simulink model "Third_Impact_final2"  (R2025a)
settings: Solver=ode23tb  StartTime=0  StopTime=1000  FixedStep=Ts  RelTol=1e-3
PostLoadFcn:
  | helperSLHighwayLaneFollowingWithRRSetup()
values from neighbouring files (symbols this model uses):
  numTargetActors = numActors - 1    [helperSLHighwayLaneFollowingWithRRSetup.m]
  vehSim3D = repmat(     struct(     'Length', 0,     'RearOverhang', 0,     'InitialPos',[0 0 0],     'InitialRot',[0 0 0]),     numVehicles,1)    [helperSLHighwayLaneFollowingWithRRSetup.m]
undefined symbols (not defined in the file or in its folder): Defined, des_vel, Ego, genDelta, genTarget, Lane, laneChange, m, n, Ts, User
libraries: sim3dautolib x5, roadrunnerscenario x4, simulink x4, sim3dlib x1
CloseFcn:
  | helperSLHighwayLaneFollowingWithRRCleanUp()
settings Model: SILPILModeSetting=veronly  SILPILSystemUnderTest=refmodels  Creator=The MathWorks, Inc.  LastModifiedBy=leskb
settings SolverCC: AlgebraicLoopSolver=TrustRegion  MaxZcPerStep=1.0
settings DataIOCC: SaveOutput=off  DSMLogging=off  SaveTime=off  ReturnWorkspaceOutputs=off
settings OptimizationCC: ReuseModelBlockBuffer=off
settings DebuggingCC: ParameterPrecisionLossMsg=none  UnconnectedInputMsg=warning  UnconnectedOutputMsg=warning  UnconnectedLineMsg=warning  PregeneratedLibrarySubsystemCodeDiagnostic=none  SubsystemReferenceDiagnosticForUnitTest=warning  ArithmeticOperatorsInVariantConditions=warning
settings HardwareCC: ProdLongLongMode=on
settings ModelReferenceCC: EnableRefExpFcnMdlSchedulingChecks=on
settings SFSimCC: SimUseLocalCustomCode=off
settings RTWCC: RTWUseLocalCustomCode=off  GPUComputeCapability=3.5  DLArmComputeVersion=19.05
settings GRTTargetCC: RTWCAPISignals=on
settings ConfigComp: CovScope=ReferencedModels  CovIncludeTopModel=off

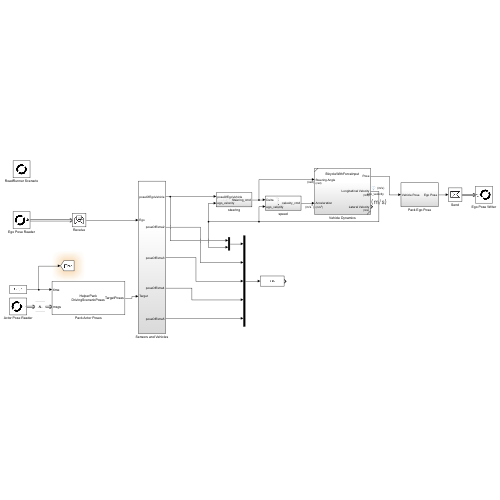
[thumbnail: Simulink's stored preview of the top-level diagram]
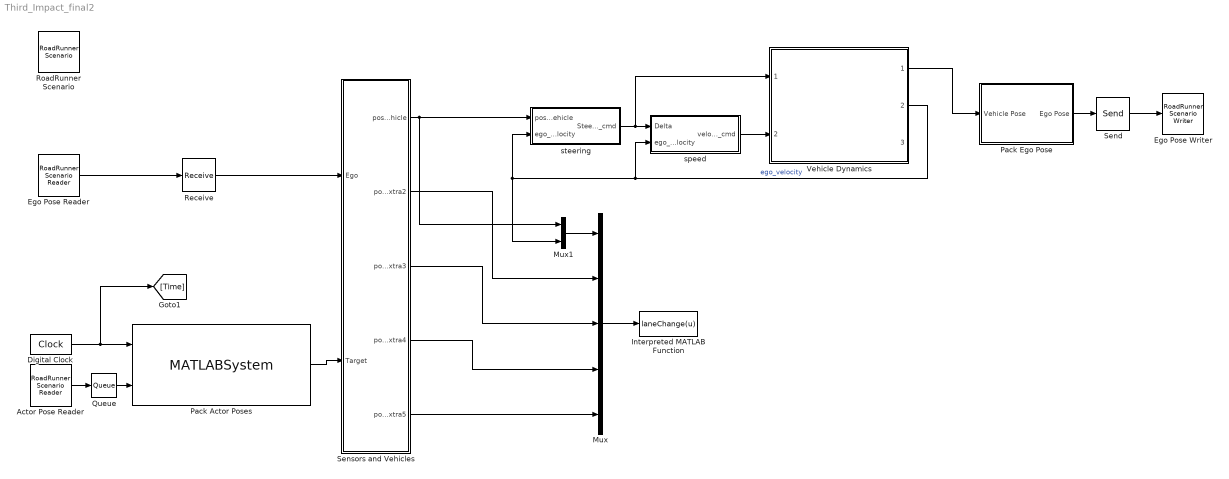
== system Third_Impact_final2 ==
  Actor Pose Reader : roadrunnerscenario/RoadRunner Scenario Reader  TopicCategory=Actor  ActorCategory=All Types  ActionType=Path Following  EventType=User-Defined  TopicType=Actor Pose (Driving Scenario compatible)  VehicleType=Vehicle Specifications  TrafficSignalType=Traffic Signal Specifications  TrafficSignalControllerType=Traffic Signal Controller Specifications  UserDefinedAction=Action1  UserDefinedEvent=Event1  Filter=None  AdditionalRelationship=None  SensorTopic=Target Poses  LaneBoundaryOutputTopic=Ego-Lane  SensorID=1  SampleTime=Ts
  Digital Clock : DigitalClock  SampleTime=Ts
  Ego Pose Reader : roadrunnerscenario/RoadRunner Scenario Reader  TopicCategory=Actor  ActorCategory=All Types  ActionType=Path Following  EventType=User-Defined  TopicType=Actor Pose (Driving Scenario compatible)  VehicleType=Vehicle Specifications  TrafficSignalType=Traffic Signal Specifications  TrafficSignalControllerType=Traffic Signal Controller Specifications  UserDefinedAction=Action1  UserDefinedEvent=Event1  Filter=Self  AdditionalRelationship=None  SensorTopic=Target Poses  LaneBoundaryOutputTopic=Ego-Lane  SensorID=1  SampleTime=Ts
  Ego Pose Writer : roadrunnerscenario/RoadRunner Scenario Writer  TopicCategory=Actor  ActorCategory=All Types  EventType=Action Complete  UserDefinedEvent=Event1  VehicleType=Vehicle Pose  TopicType=Actor Pose (Driving Scenario compatible)
  Interpreted MATLAB Function : MATLABFcn  MATLABFcn=laneChange(u)
  Mux : Mux  Inputs=[4 4 4 4 4]
  Mux1 : Mux  Inputs=2
  Pack Actor Poses : MATLABSystem  InputPortMessageModes=n,m  System=HelperPackDrivingScenarioPoses  EgoActorID=1  ActorProfiles=actorProfiles  DefaultActorPoses="Simulink.Bus.createMATLABStruct( \"BusActors\" )"
      mask Type: HelperPackDrivingScenarioPoses
  Pack Ego Pose : Subsystem
  Queue : Queue  InputPortMessageModes=m  OutputPortMessageModes=m  OverwriteOldest=on  Capacity=numTargetActors+2  QueueType=LIFO
  Receive : Receive  InputPortMessageModes=m  UseInternalQueue=off  QueueOverwriting=on  QueueLength=1  QueueType=LIFO  SampleTime=Ts
  RoadRunner Scenario : roadrunnerscenario/RoadRunner Scenario  UserDefinedActions={}  UserDefinedEvents={}  PathPoints=500
  Send : Send  OutputPortMessageModes=m
  Sensors and Vehicles : Subsystem  VariantControl=1
  Vehicle Dynamics : Subsystem  VariantControl=Variant2  ReferencedSubsystem=BicycleWithForceInput
  speed : Subsystem
  steering : Subsystem
  wires:
  Ego Pose Reader/1 -> Receive/1
  Digital Clock/1 -> Pack Actor Poses/1, [Time]
  Send/1 -> Ego Pose Writer/1
  Vehicle Dynamics/1 -> Pack Ego Pose/1(Vehicle Pose)
  Receive/1 -> Sensors and Vehicles/1(Ego)
  Actor Pose Reader/1 -> Queue/1
  Pack Ego Pose/1(Ego Pose) -> Send/1
  Queue/1 -> Pack Actor Poses/2
  Pack Actor Poses/1 -> Sensors and Vehicles/2(Target)
  Vehicle Dynamics/2 -> speed/2(ego_velocity), steering/2(ego_velocity), Mux1/2  "ego_velocity"
  speed/1(velocity_cmd) -> Vehicle Dynamics/2
  steering/1(Steering_cmd) -> speed/1(Delta), Vehicle Dynamics/1
  Sensors and Vehicles/1(poseOfEgoVehicle) -> Mux1/1, steering/1(poseOfEgoVehicle)
  Sensors and Vehicles/2(poseOfExtra2) -> Mux/2
  Sensors and Vehicles/3(poseOfExtra3) -> Mux/3
  Sensors and Vehicles/4(poseOfExtra4) -> Mux/4
  Sensors and Vehicles/5(poseOfExtra5) -> Mux/5
  Mux/1 -> Interpreted MATLAB Function/1
  Mux1/1 -> Mux/1

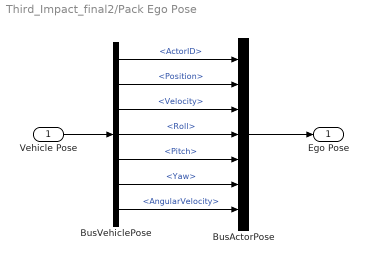
== system Third_Impact_final2/Pack Ego Pose ==
  Vehicle Pose : Inport
  BusActorPose : BusCreator  Inputs=7  OutDataTypeStr=Bus: BusActorPose  NonVirtualBus=on
      settings: InheritFromInputs=off
  BusVehiclePose : BusSelector  OutputSignals=ActorID,Position,Velocity,Roll,Pitch,Yaw,AngularVelocity
  Ego Pose : Outport
  wires:
  BusVehiclePose/4 -> BusActorPose/4  "<Roll>"
  BusVehiclePose/3 -> BusActorPose/3  "<Velocity>"
  BusVehiclePose/1 -> BusActorPose/1  "<ActorID>"
  BusVehiclePose/2 -> BusActorPose/2  "<Position>"
  BusVehiclePose/7 -> BusActorPose/7  "<AngularVelocity>"
  BusVehiclePose/6 -> BusActorPose/6  "<Yaw>"
  BusVehiclePose/5 -> BusActorPose/5  "<Pitch>"
  Vehicle Pose/1 -> BusVehiclePose/1
  BusActorPose/1 -> Ego Pose/1

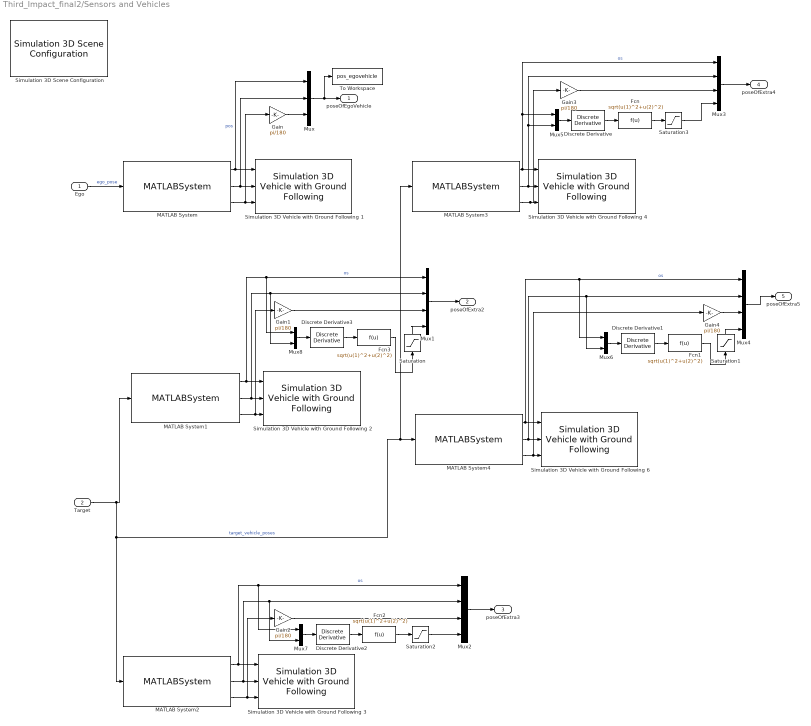
== system Third_Impact_final2/Sensors and Vehicles ==
  Ego : Inport
  Target : Inport  Port=2
  Discrete Derivative{,1..3} (4 alike) : simulink/Discrete/Discrete Derivative  gainval=1.0  ICPrevScaledInput=0.0  OutMin=[]  OutMax=[]  OutDataType=fixdt(1, 16)  OutScaling=2^-10  DoSatur=off
  Fcn{,1..3} (4 alike) : Fcn  Expr=sqrt(u(1)^2+u(2)^2)
  Gain{,1..4} (5 alike) : Gain  Gain=pi/180
  MATLAB System : MATLABSystem  System=HelperConvertDSPoseToSim3D  ActorProfiles=actorProfiles  ActorIDToConvert=1  SimulateUsing=Interpreted execution
      mask Type: HelperConvertDSPoseToSim3D
  MATLAB System1 : MATLABSystem  System=HelperConvertDSPoseToSim3D  ActorProfiles=actorProfiles  ActorIDToConvert=2  SimulateUsing=Interpreted execution
      mask Type: HelperConvertDSPoseToSim3D
  MATLAB System2 : MATLABSystem  System=HelperConvertDSPoseToSim3D  ActorProfiles=actorProfiles  ActorIDToConvert=3  SimulateUsing=Interpreted execution
      mask Type: HelperConvertDSPoseToSim3D
  MATLAB System3 : MATLABSystem  System=HelperConvertDSPoseToSim3D  ActorProfiles=actorProfiles  ActorIDToConvert=4  SimulateUsing=Interpreted execution
      mask Type: HelperConvertDSPoseToSim3D
  MATLAB System4 : MATLABSystem  System=HelperConvertDSPoseToSim3D  ActorProfiles=actorProfiles  ActorIDToConvert=5  SimulateUsing=Interpreted execution
      mask Type: HelperConvertDSPoseToSim3D
  Mux : Mux  Inputs=3
  Mux{1..4} (4 alike) : Mux
  Mux{5..8} (4 alike) : Mux  Inputs=2
  Saturation{,1..3} (4 alike) : Saturate  UpperLimit=100  LowerLimit=-100
  Simulation 3D Scene Configuration : sim3dlib/Simulation 3D Scene Configuration  Priority=0  ProjectFormat=Default Scenes  SceneDesc=Straight road  ProjectName=C:\Program Files\MATLAB\R2025a\toolbox\shared\sim3d_projects\automotive_project_windows\UE\WindowsNoEditor\VehicleSimulation.exe  ScenePath=/Game/Maps/HwStrght  EnableOpenDRIVE=off  vehTagList={'Custom';'Scene Origin';'SimulinkVehicle1';'SimulinkVehicle2';'SimulinkVehicle4';'SimulinkVehicle5';'SimulinkVehicle6'}  vehTag=SimulinkVehicle1  AttachedCameraRelativeTranslation=[0 0 0]  FreeCameraDefaultInitialTranslation=[-6, 0, 2]  AttachedCameraRelativeRotation=[0 0 0]  FreeCameraDefaultInitialRotation=[0, -15, 0]  ViewpointName=Custom  FreeCameraInitialTranslation=[0, 0, 0]  ViewpointTranslation=[0 0 0]  FreeCameraInitialRotation=[0, 0, 0]  ViewpointRotation=[0 0 0]  OpVisEn=off  Ts=Ts  EnableWindow=off  EnableRemoteAccess=off  EnableWeather=off  SunAzimuth=90  SunAltitude=40.0  EnableGeospatialSun=off  Latitude=0  Longitude=0  Date=2023-01-01  Time=10:30:00  GeoTimeZone=-5.0  SunDaylightSaving=off  wind=1  clouds=10  EnableVolumetricClouds=off  CloudCoverage=0  CloudAltitude=6  fog=0  rain=0  RaindropsEffect=off  SnowDensity=0  EnableGeospatial=off  TilesetSource=Earth terrain  UseTrueOrigin=off  OriginHeight=200  OriginLatitude=40.744652  OriginLongitude=-73.988864  MapStyle=Aerial  AdditionalAssetIDs=[]  UseAdvancedSunSky=off  SolarTime=11  TimeZone=-5  Day=21  Month=9  Year=2022  UseDaylightSavingTime=on  DSTStartDay=10  DSTStartMonth=3  DSTEndDay=3  DSTEndMonth=11  DSTSwitchHour=2  sensorTag=MainCamera3  sensorId=3  sensorName=MainCamera3  mountLoc=Origin  offsetFlag=off  tmountOffset=[0, 0, 0]  rmountOffset=[0, 0, 0]  HorizontalResolution=1280  VerticalResolution=720  HorizontalFOV=60  mountPoint=[0 0 0]  mountOrientation=[0 0 0]  aMode=3  ID=3  GeoTrigger=Inactive  ViewNameList={'Custom'}  ViewTranslationList={'[0 0 0]'}  ViewRotationList={'[0 0 0]'}
      settings: LibrarySourceBlock=drivingsim3d/Simulation 3D Scene Configuration
  Simulation 3D Vehicle with Ground Following 1 : sim3dautolib/Simulation 3D Vehicle with Ground Following  Priority=-1  PassVehMesh=Sedan  MeshPath=/MathWorksSimulation/Vehicles/Muscle/Meshes/SK_MuscleCar.SK_MuscleCar  TrackWidth=1.9  WheelBase=3  WheelRadius=0.35  VehColor=Blue  CoordinateSystem=ISO8855  InitialPos=vehSim3D(1).InitialPos  InitialRot=vehSim3D(1).InitialRot  ActorName=SimulinkVehicle1  SampleTime=-1  ActorType=SimulinkVehicle  ID=1  aMode=3  ActorTag=SimulinkVehicle1  CoordinateScheme=ISO  VehLightsControl=off  HeadlightColor=[ 1, 1, 1 ]  HighBeamIntensity=100000  LowBeamIntensity=60000  HighBeamConeAngle=70  LowBeamConeAngle=70  LeftHeadlightOrientation=[ 0, 0 ]  RightHeadlightOrientation=[ 0, 0 ]  BrakelightIntensity=500  ReverselightIntensity=500  SignallightIntensity=500  SignallightPeriod=1  SignalPulseWidth=50  TransformOutportEnabled=off
      settings: LibrarySourceBlock=drivingsim3d/Simulation 3D Vehicle with Ground Following
      settings: AttributesFormatString=|
      | --------------------------------------
      | ActorName = %<ActorName>
      | PassVehMesh = %<PassVehMesh>
      | VehColor = %<VehColor>
      | InitialPos = %<InitialPos>
      | InitialRot = %<InitialRot>
      | Priority = %<Priority>
  Simulation 3D Vehicle with Ground Following 2 : sim3dautolib/Simulation 3D Vehicle with Ground Following  Priority=-1  PassVehMesh=Sedan  MeshPath=/MathWorksSimulation/Vehicles/Muscle/Meshes/SK_MuscleCar.SK_MuscleCar  TrackWidth=1.9  WheelBase=3  WheelRadius=0.35  VehColor=Red  CoordinateSystem=ISO8855  InitialPos=vehSim3D(2).InitialPos  InitialRot=vehSim3D(2).InitialRot  ActorName=SimulinkVehicle2  SampleTime=-1  ActorType=SimulinkVehicle  ID=2  aMode=3  ActorTag=SimulinkVehicle2  CoordinateScheme=ISO  VehLightsControl=off  HeadlightColor=[ 1, 1, 1 ]  HighBeamIntensity=100000  LowBeamIntensity=60000  HighBeamConeAngle=70  LowBeamConeAngle=70  LeftHeadlightOrientation=[ 0, 0 ]  RightHeadlightOrientation=[ 0, 0 ]  BrakelightIntensity=500  ReverselightIntensity=500  SignallightIntensity=500  SignallightPeriod=1  SignalPulseWidth=50  TransformOutportEnabled=off
      settings: LibrarySourceBlock=drivingsim3d/Simulation 3D Vehicle with Ground Following
      settings: AttributesFormatString=|
      | --------------------------------------
      | ActorName = %<ActorName>
      | PassVehMesh = %<PassVehMesh>
      | VehColor = %<VehColor>
      | InitialPos = %<InitialPos>
      | InitialRot = %<InitialRot>
      | Priority = %<Priority>
  Simulation 3D Vehicle with Ground Following 3 : sim3dautolib/Simulation 3D Vehicle with Ground Following  Priority=-1  PassVehMesh=Sedan  MeshPath=/MathWorksSimulation/Vehicles/Muscle/Meshes/SK_MuscleCar.SK_MuscleCar  TrackWidth=1.9  WheelBase=3  WheelRadius=0.35  VehColor=Black  CoordinateSystem=ISO8855  InitialPos=vehSim3D(3).InitialPos  InitialRot=vehSim3D(3).InitialRot  ActorName=SimulinkVehicle4  SampleTime=-1  ActorType=SimulinkVehicle  ID=4  aMode=3  ActorTag=SimulinkVehicle4  CoordinateScheme=ISO  VehLightsControl=off  HeadlightColor=[ 1, 1, 1 ]  HighBeamIntensity=100000  LowBeamIntensity=60000  HighBeamConeAngle=70  LowBeamConeAngle=70  LeftHeadlightOrientation=[ 0, 0 ]  RightHeadlightOrientation=[ 0, 0 ]  BrakelightIntensity=500  ReverselightIntensity=500  SignallightIntensity=500  SignallightPeriod=1  SignalPulseWidth=50  TransformOutportEnabled=off
      settings: LibrarySourceBlock=drivingsim3d/Simulation 3D Vehicle with Ground Following
      settings: AttributesFormatString=|
      | --------------------------------------
      | ActorName = %<ActorName>
      | PassVehMesh = %<PassVehMesh>
      | VehColor = %<VehColor>
      | InitialPos = %<InitialPos>
      | InitialRot = %<InitialRot>
      | Priority = %<Priority>
  Simulation 3D Vehicle with Ground Following 4 : sim3dautolib/Simulation 3D Vehicle with Ground Following  Priority=-1  PassVehMesh=Sedan  MeshPath=/MathWorksSimulation/Vehicles/Muscle/Meshes/SK_MuscleCar.SK_MuscleCar  TrackWidth=1.9  WheelBase=3  WheelRadius=0.35  VehColor=Orange  CoordinateSystem=ISO8855  InitialPos=vehSim3D(4).InitialPos  InitialRot=vehSim3D(4).InitialRot  ActorName=SimulinkVehicle5  SampleTime=-1  ActorType=SimulinkVehicle  ID=5  aMode=3  ActorTag=SimulinkVehicle5  CoordinateScheme=ISO  VehLightsControl=off  HeadlightColor=[ 1, 1, 1 ]  HighBeamIntensity=100000  LowBeamIntensity=60000  HighBeamConeAngle=70  LowBeamConeAngle=70  LeftHeadlightOrientation=[ 0, 0 ]  RightHeadlightOrientation=[ 0, 0 ]  BrakelightIntensity=500  ReverselightIntensity=500  SignallightIntensity=500  SignallightPeriod=1  SignalPulseWidth=50  TransformOutportEnabled=off
      settings: LibrarySourceBlock=drivingsim3d/Simulation 3D Vehicle with Ground Following
      settings: AttributesFormatString=|
      | --------------------------------------
      | ActorName = %<ActorName>
      | PassVehMesh = %<PassVehMesh>
      | VehColor = %<VehColor>
      | InitialPos = %<InitialPos>
      | InitialRot = %<InitialRot>
      | Priority = %<Priority>
  Simulation 3D Vehicle with Ground Following 6 : sim3dautolib/Simulation 3D Vehicle with Ground Following  Priority=-1  PassVehMesh=Sedan  MeshPath=/MathWorksSimulation/Vehicles/Muscle/Meshes/SK_MuscleCar.SK_MuscleCar  TrackWidth=1.9  WheelBase=3  WheelRadius=0.35  VehColor=Green  CoordinateSystem=ISO8855  InitialPos=vehSim3D(5).InitialPos  InitialRot=vehSim3D(5).InitialRot  ActorName=SimulinkVehicle6  SampleTime=-1  ActorType=SimulinkVehicle  ID=6  aMode=3  ActorTag=SimulinkVehicle6  CoordinateScheme=ISO  VehLightsControl=off  HeadlightColor=[ 1, 1, 1 ]  HighBeamIntensity=100000  LowBeamIntensity=60000  HighBeamConeAngle=70  LowBeamConeAngle=70  LeftHeadlightOrientation=[ 0, 0 ]  RightHeadlightOrientation=[ 0, 0 ]  BrakelightIntensity=500  ReverselightIntensity=500  SignallightIntensity=500  SignallightPeriod=1  SignalPulseWidth=50  TransformOutportEnabled=off
      settings: LibrarySourceBlock=drivingsim3d/Simulation 3D Vehicle with Ground Following
      settings: AttributesFormatString=|
      | --------------------------------------
      | ActorName = %<ActorName>
      | PassVehMesh = %<PassVehMesh>
      | VehColor = %<VehColor>
      | InitialPos = %<InitialPos>
      | InitialRot = %<InitialRot>
      | Priority = %<Priority>
  To Workspace : ToWorkspace  VariableName=pos_egovehicle  SaveFormat=Timeseries  SampleTime=-1
  poseOfEgoVehicle : Outport
  poseOfExtra2 : Outport  Port=2
  poseOfExtra3 : Outport  Port=3
  poseOfExtra4 : Outport  Port=4
  poseOfExtra5 : Outport  Port=5
  wires:
  MATLAB System/2 -> Mux/2, Simulation 3D Vehicle with Ground Following 1/2
  MATLAB System/1 -> Mux/1, Simulation 3D Vehicle with Ground Following 1/1  "pos"
  MATLAB System/3 -> Gain/1, Simulation 3D Vehicle with Ground Following 1/3
  Ego/1 -> MATLAB System/1  "ego_pose"
  Target/1 -> MATLAB System2/1, MATLAB System4/1, MATLAB System3/1, MATLAB System1/1  "target_vehicle_poses"
  Mux/1 -> To Workspace/1, poseOfEgoVehicle/1
  Gain/1 -> Mux/3
  Gain1/1 -> Mux1/3
  Mux1/1 -> poseOfExtra2/1
  MATLAB System1/3 -> Gain1/1, Simulation 3D Vehicle with Ground Following 2/3
  MATLAB System2/3 -> Gain2/1, Simulation 3D Vehicle with Ground Following 3/3
  Gain2/1 -> Mux2/3
  Mux2/1 -> poseOfExtra3/1
  MATLAB System3/3 -> Gain3/1, Simulation 3D Vehicle with Ground Following 4/3
  MATLAB System3/1 -> Mux5/1, Mux3/1, Simulation 3D Vehicle with Ground Following 4/1  "os"
  Mux3/1 -> poseOfExtra4/1
  Gain3/1 -> Mux3/3
  MATLAB System3/2 -> Mux5/2, Mux3/2, Simulation 3D Vehicle with Ground Following 4/2
  Gain4/1 -> Mux4/3
  Mux4/1 -> poseOfExtra5/1
  MATLAB System4/3 -> Gain4/1, Simulation 3D Vehicle with Ground Following 6/3
  MATLAB System4/2 -> Mux4/2, Mux6/2, Simulation 3D Vehicle with Ground Following 6/2
  Mux5/1 -> Discrete Derivative/1
  Discrete Derivative/1 -> Fcn/1
  Fcn/1 -> Saturation3/1
  Mux6/1 -> Discrete Derivative1/1
  Discrete Derivative1/1 -> Fcn1/1
  MATLAB System4/1 -> Mux4/1, Mux6/1, Simulation 3D Vehicle with Ground Following 6/1  "os"
  Fcn1/1 -> Saturation1/1
  MATLAB System2/2 -> Mux7/2, Mux2/2, Simulation 3D Vehicle with Ground Following 3/2
  Mux7/1 -> Discrete Derivative2/1
  Discrete Derivative2/1 -> Fcn2/1
  MATLAB System2/1 -> Mux7/1, Mux2/1, Simulation 3D Vehicle with Ground Following 3/1  "os"
  Fcn2/1 -> Saturation2/1
  MATLAB System1/2 -> Mux1/2, Mux8/2, Simulation 3D Vehicle with Ground Following 2/2
  Mux8/1 -> Discrete Derivative3/1
  Discrete Derivative3/1 -> Fcn3/1
  MATLAB System1/1 -> Mux8/1, Mux1/1, Simulation 3D Vehicle with Ground Following 2/1  "os"
  Fcn3/1 -> Saturation/1
  Saturation/1 -> Mux1/4
  Saturation1/1 -> Mux4/4
  Saturation2/1 -> Mux2/4
  Saturation3/1 -> Mux3/4

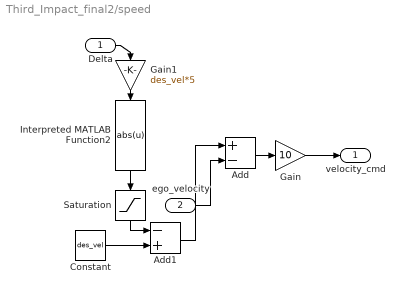
== system Third_Impact_final2/speed ==
  Delta : Inport
  ego_velocity : Inport  Port=2
  Add : Sum  Inputs=+-
  Add1 : Sum  Inputs=-+
  Constant : Constant  Value=des_vel  SampleTime=Ts
  Gain : Gain  Gain=10
  Gain1 : Gain  Gain=des_vel*5
  Interpreted MATLAB Function2 : MATLABFcn  MATLABFcn=abs(u)  OutputSignalType=real  Output1D=off
  Saturation : Saturate  UpperLimit=des_vel*0.8  LowerLimit=0
  velocity_cmd : Outport
  wires:
  Gain1/1 -> Interpreted MATLAB Function2/1
  Add/1 -> Gain/1
  Constant/1 -> Add1/2
  Delta/1 -> Gain1/1
  Saturation/1 -> Add1/1
  ego_velocity/1 -> Add/2
  Interpreted MATLAB Function2/1 -> Saturation/1
  Add1/1 -> Add/1
  Gain/1 -> velocity_cmd/1

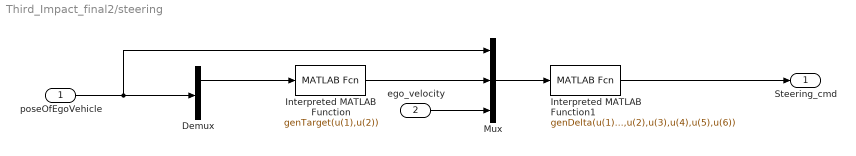
== system Third_Impact_final2/steering ==
  poseOfEgoVehicle : Inport
  ego_velocity : Inport  Port=2
  Demux : Demux  Outputs=[2 1]
  Interpreted MATLAB Function : MATLABFcn  MATLABFcn=genTarget(u(1),u(2))  OutputSignalType=real  Output1D=off
  Interpreted MATLAB Function1 : MATLABFcn  MATLABFcn=genDelta(u(1),u(2),u(3),u(4),u(5),u(6))  OutputSignalType=real  Output1D=off
  Mux : Mux  Inputs=[3 2 1]
  Steering_cmd : Outport
  wires:
  Interpreted MATLAB Function1/1 -> Steering_cmd/1
  poseOfEgoVehicle/1 -> Mux/1, Demux/1
  Mux/1 -> Interpreted MATLAB Function1/1
  ego_velocity/1 -> Mux/3
  Interpreted MATLAB Function/1 -> Mux/2
  Demux/1 -> Interpreted MATLAB Function/1
